simulink model "ramp01"  (R2023b)
settings: Solver=VariableStepAuto  StartTime=0.0  StopTime=10.0  RelTol=1e-3
libraries: simulink x4
settings Model: Creator=reemb  LastModifiedBy=reemb

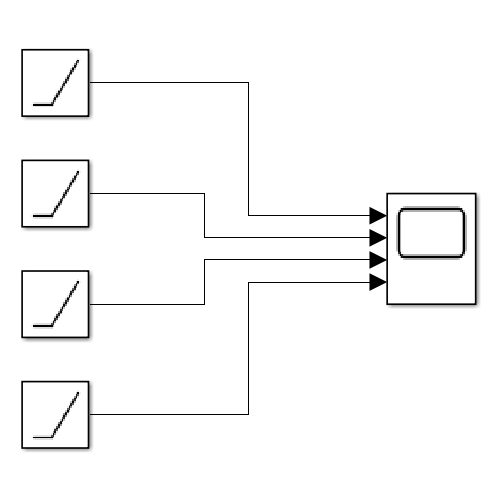
[thumbnail: Simulink's stored preview of the top-level diagram]
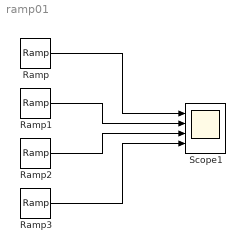
== system ramp01 ==
  Ramp : simulink/Sources/Ramp  slope=1  start=0  InitialOutput=0
  Ramp1 : simulink/Sources/Ramp  slope=1  start=1  InitialOutput=0
  Ramp2 : simulink/Sources/Ramp  slope=1  start=5  InitialOutput=0
  Ramp3 : simulink/Sources/Ramp  slope=1  start=5  InitialOutput=1
  Scope1 : Scope  NumInputPorts=4
  wires:
  Ramp/1 -> Scope1/1
  Ramp1/1 -> Scope1/2
  Ramp2/1 -> Scope1/3
  Ramp3/1 -> Scope1/4
